simulink model "Six_phase_inverter_twoThree_pwm"  (R2014b)
settings: Solver=ode23tb  StartTime=0.0  StopTime=0.05  MaxStep=1e-4  RelTol=1e-3
InitFcn:
  | Vm=0.5;
  | Fc=3000;
libraries: powerlib x12, powerlib_meascontrol x2
settings Model: Creator=y  LastModifiedBy=Lei
settings DataIOCC: SignalLoggingSaveFormat=ModelDataLogs
settings OptimizationCC: ExpressionDepthLimit=2147483647  InitFltsAndDblsToZero=on
settings DebuggingCC: SaveWithParameterizedLinksMsg=none  UnderspecifiedInitializationDetection=Classic  MergeDetectMultiDrivingBlocksExec=none  SignalResolutionControl=TryResolveAllWithWarning  MultiTaskDSMMsg=warning  MultiTaskCondExecSysMsg=none  FcnCallInpInsideContextMsg=UseLocalSettings  StateNameClashWarn=warning
settings RTWCC: IncludeERTFirstTime=on
settings GRTTargetCC: TargetFcnLib=ansi_tfl_tmw.mat  CombineOutputUpdateFcns=off  GRTInterface=on

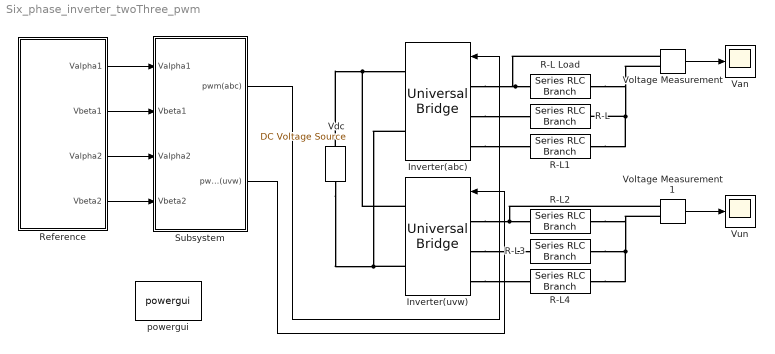
== system Six_phase_inverter_twoThree_pwm ==
  Inverter(abc) : powerlib/Power Electronics/Universal Bridge  Arms=3  SnubberResistance=1e5  SnubberCapacitance=inf  Device=IGBT / Diodes  Ron=1e-3  Lon=0  ForwardVoltages="[  0  0  ]"  ForwardVoltage=0  GTOparameters=[ 10e-6 , 20e-6 ]  IGBTparameters=[ 1e-6 , 2e-6 ]  Measurements=None  Measurements_2=None  converterType=Rectifier
  Inverter(uvw) : powerlib/Power Electronics/Universal Bridge  Arms=3  SnubberResistance=1e5  SnubberCapacitance=inf  Device=IGBT / Diodes  Ron=1e-3  Lon=0  ForwardVoltages="[  0  0  ]"  ForwardVoltage=0  GTOparameters=[ 10e-6 , 20e-6 ]  IGBTparameters=[ 1e-6 , 2e-6 ]  Measurements=None  Measurements_2=None  converterType=Rectifier
  R-L{,1..4} (5 alike) : powerlib/Elements/Series RLC Branch  LConnTagsString=__new0  RConnTagsString=__new0  BranchType=RL  Resistance=10  Inductance=1e-03  SetiL0=off  InitialCurrent=0  Capacitance=[]  Setx0=off  InitialVoltage=0  Measurements=None
  R-L Load : powerlib/Elements/Series RLC Branch  LConnTagsString=__new0  RConnTagsString=__new0  BranchType=RL  Resistance=10  Inductance=1e-03  SetiL0=off  InitialCurrent=0  Capacitance=[]  Setx0=off  InitialVoltage=0  Measurements=None
  Reference : Subsystem
      mask Display:
      | disp('reference\nvoltage\ngenerator')
      | port_label('output',1,'Valpha1')
      | port_label('output',2,'Vbeta1')
      | port_label('output',3,'Valpha2')
      | port_label('output',4,'Vbeta2')
  Subsystem : Subsystem
  Van : Scope
      settings: TimeRange=0.05  YMin=-200  YMax=200  SaveName=Van  SampleInput=on  SampleTime=1e-6
  Vdc : powerlib/Electrical Sources/DC Voltage Source  Amplitude=300  Measurements=None
  Voltage Measurement : powerlib/Measurements/Voltage Measurement  PhasorSimulation=off  OutputType=Complex  PSBequivalent=0
  Voltage Measurement1 : powerlib/Measurements/Voltage Measurement  PhasorSimulation=off  OutputType=Complex  PSBequivalent=0
  Vun : Scope
      settings: YMin=-200  YMax=200  SaveName=Vbn  SampleInput=on  SampleTime=1e-6
  powergui : powerlib/powergui  Priority=1  SimulationMode=Continuous  SolverType=Tustin/Backward Euler (TBE)  SampleTime=50e-6  frequency=60  SPID=off  DisableSnubberDevices=off  DisableRonSwitches=off  DisableVfSwitches=off  SwTol=0  DisplayEquations=off  Interpol=off  methode=off  Ts=100  frequencyindice=0  Pbase=100e6  ErrMax=1e-4  Iterations=50  UnitsV=kV  UnitsW=MW  FunctionMessages=off  echomessages=off  HookPort=off  EnableUseOfTLC=off  x0status=blocks  RestoreLinks=warning  ResistiveCurrentMeasurement=off  Frange=[0:2:500]  Ylog=off  Xlog=on  ShowGrid=off  save=off  variable=ZData  structure=0  ZoomFFT=off  StartTime=0.0  cycles=1  DisplayStyle=1  fundamental=60  FreqAxis=off  MaxFrequency=1000  frequencyindicesteady=1  RmsSteady=1  display=off
  wires:
  Voltage Measurement/1 -> Van/1
  Voltage Measurement1/1 -> Vun/1
  Subsystem/1(pwm(abc)) -> Inverter(abc)/1
  Subsystem/2(pwm(uvw)) -> Inverter(uvw)/1
  Reference/1(Valpha1) -> Subsystem/1(Valpha1)
  Reference/2(Vbeta1) -> Subsystem/2(Vbeta1)
  Reference/3(Valpha2) -> Subsystem/3(Valpha2)
  Reference/4(Vbeta2) -> Subsystem/4(Vbeta2)
  connections:
  R-L Load/LConn1 -- Inverter(abc)/LConn1 -- Voltage Measurement/LConn1
  Inverter(abc)/LConn2 -- R-L/LConn1
  Inverter(abc)/LConn3 -- R-L1/LConn1
  Voltage Measurement1/LConn1 -- Inverter(uvw)/LConn1 -- R-L2/LConn1
  Inverter(uvw)/LConn2 -- R-L3/LConn1
  Inverter(uvw)/LConn3 -- R-L4/LConn1
  R-L4/RConn1 -- Voltage Measurement1/LConn2 -- R-L2/RConn1 -- R-L3/RConn1
  R-L1/RConn1 -- Voltage Measurement/LConn2 -- R-L Load/RConn1 -- R-L/RConn1
  Vdc/RConn1 -- Inverter(uvw)/RConn1 -- Inverter(abc)/RConn1
  Vdc/LConn1 -- Inverter(uvw)/RConn2 -- Inverter(abc)/RConn2

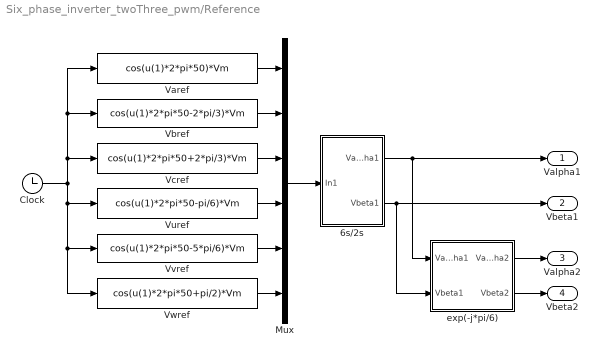
== system Six_phase_inverter_twoThree_pwm/Reference ==
  6s/2s : Subsystem
  Clock : Clock
  Mux : Mux  Inputs=6
  Varef : Fcn  Expr=cos(u(1)*2*pi*50)*Vm
  Vbref : Fcn  Expr=cos(u(1)*2*pi*50-2*pi/3)*Vm
  Vcref : Fcn  Expr=cos(u(1)*2*pi*50+2*pi/3)*Vm
  Vuref : Fcn  Expr=cos(u(1)*2*pi*50-pi/6)*Vm
  Vvref : Fcn  Expr=cos(u(1)*2*pi*50-5*pi/6)*Vm
  Vwref : Fcn  Expr=cos(u(1)*2*pi*50+pi/2)*Vm
  exp(-j*pi/6) : Subsystem
  Valpha1 : Outport
  Vbeta1 : Outport  Port=2
  Valpha2 : Outport  Port=3
  Vbeta2 : Outport  Port=4
  wires:
  Varef/1 -> Mux/1
  Clock/1 -> Varef/1, Vbref/1, Vcref/1, Vwref/1, Vvref/1, Vuref/1
  Vbref/1 -> Mux/2
  Vcref/1 -> Mux/3
  Vvref/1 -> Mux/5
  Vwref/1 -> Mux/6
  Vuref/1 -> Mux/4
  6s/2s/1(Valpha1) -> Valpha1/1, exp(-j*pi/6)/1(Valpha1)
  6s/2s/2(Vbeta1) -> exp(-j*pi/6)/2(Vbeta1), Vbeta1/1
  Mux/1 -> 6s/2s/1(In1)
  exp(-j*pi/6)/1(Valpha2) -> Valpha2/1
  exp(-j*pi/6)/2(Vbeta2) -> Vbeta2/1

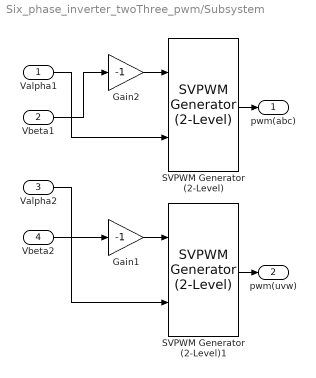
== system Six_phase_inverter_twoThree_pwm/Subsystem ==
  Valpha1 : Inport
  Vbeta1 : Inport  Port=2
  Valpha2 : Inport  Port=3
  Vbeta2 : Inport  Port=4
  Gain1 : Gain  Gain=-1
  Gain2 : Gain  Gain=-1
  SVPWM Generator (2-Level) : powerlib_meascontrol/Pulse & Signal Generators/SVPWM Generator (2-Level)  InputType=alpha-beta components  SwitchingPattern=Pattern #1  Fc=5000  ParUref=[0.8 -30 50]  Ts=0
  SVPWM Generator (2-Level)1 : powerlib_meascontrol/Pulse & Signal Generators/SVPWM Generator (2-Level)  InputType=alpha-beta components  SwitchingPattern=Pattern #1  Fc=5000  ParUref=[0.8 -30 50]  Ts=0
  pwm(abc) : Outport
  pwm(uvw) : Outport  Port=2
  wires:
  Gain1/1 -> SVPWM Generator (2-Level)1/1
  Vbeta2/1 -> Gain1/1
  Valpha2/1 -> SVPWM Generator (2-Level)1/2
  SVPWM Generator (2-Level)1/1 -> pwm(uvw)/1
  SVPWM Generator (2-Level)/1 -> pwm(abc)/1
  Vbeta1/1 -> Gain2/1
  Valpha1/1 -> SVPWM Generator (2-Level)/2
  Gain2/1 -> SVPWM Generator (2-Level)/1

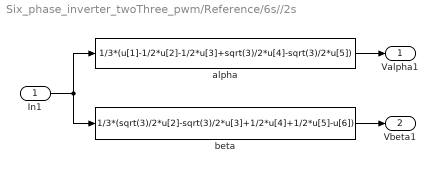
== system Six_phase_inverter_twoThree_pwm/Reference/6s//2s ==
  In1 : Inport
  alpha : Fcn  Expr=1/3*(u[1]-1/2*u[2]-1/2*u[3]+sqrt(3)/2*u[4]-sqrt(3)/2*u[5])
  beta : Fcn  Expr=1/3*(sqrt(3)/2*u[2]-sqrt(3)/2*u[3]+1/2*u[4]+1/2*u[5]-u[6])
  Valpha1 : Outport
  Vbeta1 : Outport  Port=2
  wires:
  In1/1 -> alpha/1, beta/1
  alpha/1 -> Valpha1/1
  beta/1 -> Vbeta1/1

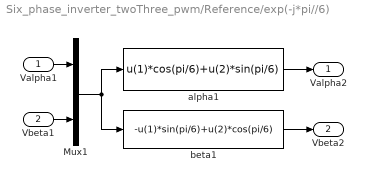
== system Six_phase_inverter_twoThree_pwm/Reference/exp(-j*pi//6) ==
  Valpha1 : Inport
  Vbeta1 : Inport  Port=2
  Mux1 : Mux  Inputs=2
  alpha1 : Fcn  Expr=u(1)*cos(pi/6)+u(2)*sin(pi/6)
  beta1 : Fcn  Expr=-u(1)*sin(pi/6)+u(2)*cos(pi/6)
  Valpha2 : Outport
  Vbeta2 : Outport  Port=2
  wires:
  beta1/1 -> Vbeta2/1
  Mux1/1 -> beta1/1, alpha1/1
  Vbeta1/1 -> Mux1/2
  Valpha1/1 -> Mux1/1
  alpha1/1 -> Valpha2/1
